simulink model "car_pid"  (Simulink 8.9)
settings: Solver=VariableStepAuto  StartTime=0.0  StopTime=15  RelTol=1e-3
settings Model: Creator=dai.490  LastModifiedBy=dai.490
settings DataIOCC: LimitDataPoints=off  SaveFormat=Dataset  SignalLoggingSaveFormat=Dataset
settings OptimizationCC: LifeSpan=auto
settings DebuggingCC: UnderspecifiedInitializationDetection=Simplified  MergeDetectMultiDrivingBlocksExec=error  FcnCallInpInsideContextMsg=error  StateNameClashWarn=none  SFUnexpectedBacktrackingDiag=error  SFNoUnconditionalDefaultTransitionDiag=error  SFExecutionAtInitializationDiag=warning
settings HardwareCC: ProdBitPerPointer=64  ProdBitPerSizeT=64  ProdBitPerPtrDiffT=64  ProdLargestAtomicFloat=Float  ProdIntDivRoundTo=Zero  ProdEndianess=LittleEndian  ProdWordSize=64  ProdHWDeviceType=Intel->x86-64 (Windows64)
settings ModelReferenceCC: PropagateSignalLabelsOutOfModel=on
settings GRTTargetCC: TargetLangStandard=C99 (ISO)  GeneratePreprocessorConditionals=Use local settings  CombineOutputUpdateFcns=on  GRTInterface=off
settings ConfigComp: CovMetricSettings=dwe  CovHtmlReporting=off  CovSaveCumulativeToWorkspaceVar=off  CovSaveSingleToWorkspaceVar=off  CovExternalEMLEnable=on

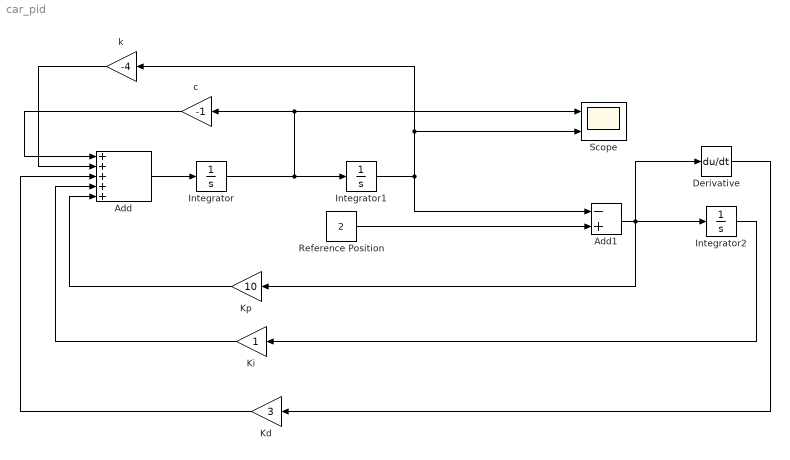
== system car_pid ==
  Add : Sum  Inputs=+++++
  Add1 : Sum  Inputs=-+
  Derivative : Derivative
  Integrator : Integrator  AbsoluteTolerance=1e-9
  Integrator1 : Integrator  AbsoluteTolerance=1e-9
  Integrator2 : Integrator  InitialCondition=0.4  AbsoluteTolerance=1e-9
  Kd : Gain  Gain=3
  Ki : Gain
  Kp : Gain  Gain=10
  Reference Position : Constant  Value=2
  Scope : Scope  NumInputPorts=2
  c : Gain  Gain=-1
  k : Gain  Gain=-4
  wires:
  k/1 -> Add/2
  Integrator/1 -> c/1, Scope/1, Integrator1/1
  Integrator1/1 -> Add1/1, Scope/2, k/1
  c/1 -> Add/1
  Add/1 -> Integrator/1
  Reference Position/1 -> Add1/2
  Add1/1 -> Derivative/1, Integrator2/1, Kp/1
  Integrator2/1 -> Ki/1
  Kp/1 -> Add/5
  Derivative/1 -> Kd/1
  Ki/1 -> Add/4
  Kd/1 -> Add/3
